simulink model "cp_2_10_Andrew_Cox"  (R2021a)
settings: Solver=VariableStepAuto  StartTime=0.0  StopTime=10.0  RelTol=1e-3
settings Model: Creator=Reaper124  LastModifiedBy=Reaper124

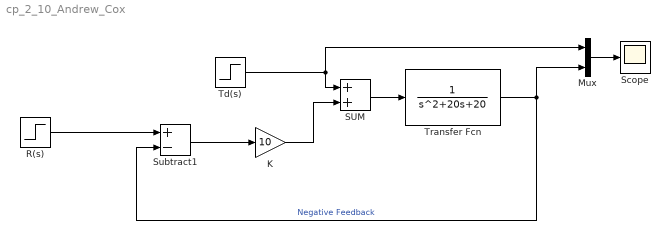
== system cp_2_10_Andrew_Cox ==
  K : Gain  Gain=10
  Mux : Mux  Inputs=2
  R(s) : Step  Time=0.1  SampleTime=0
  SUM : Sum
  Scope : Scope
  Subtract1 : Sum  Inputs=+-
  Td(s) : Step  SampleTime=0
  Transfer Fcn : TransferFcn  Denominator=[1 20 20]
  wires:
  K/1 -> SUM/2
  SUM/1 -> Transfer Fcn/1
  Subtract1/1 -> K/1
  Transfer Fcn/1 -> Mux/2, Subtract1/2  "Negative Feedback"
  R(s)/1 -> Subtract1/1
  Td(s)/1 -> SUM/1, Mux/1
  Mux/1 -> Scope/1
